simulink model "PB"  (R2025b)
settings: Solver=FixedStepAuto  StartTime=0.0  StopTime=inf  FixedStep=1E-2  RelTol=1e-3
libraries: aerolibanimutils x1
settings Model: Creator=abstract  LastModifiedBy=abstract

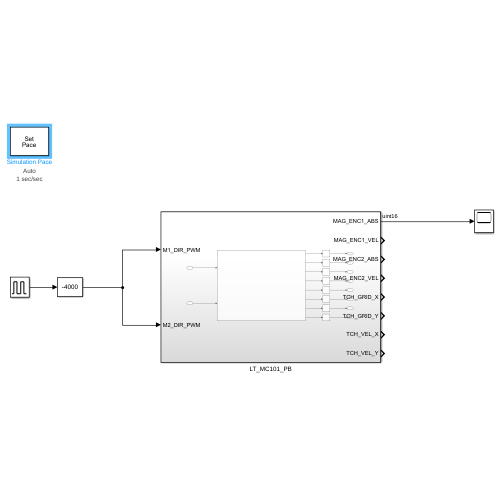
[thumbnail: Simulink's stored preview of the top-level diagram]
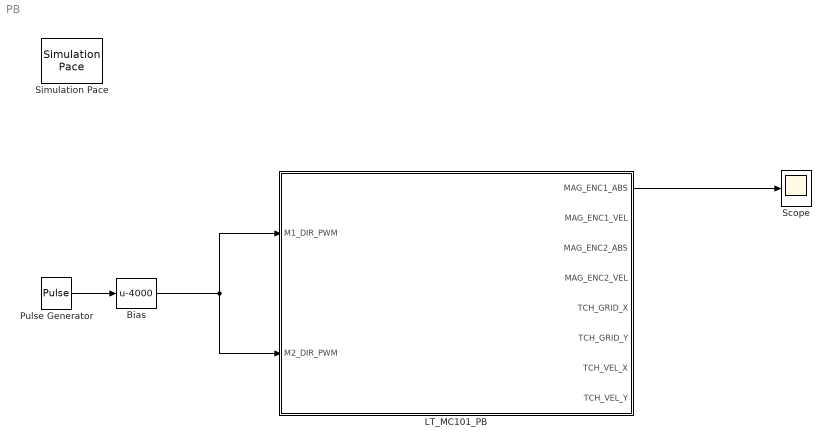
== system PB ==
  Bias : Bias  Bias=-4000  SaturateOnIntegerOverflow=off
  LT_MC101_PB : Subsystem
  Pulse Generator : DiscretePulseGenerator  PulseType=Time based  Amplitude=8000  Period=1  PulseWidth=50
  Scope : Scope
      settings: ActiveDisplayYMinimum=-62.499999999999986  ActiveDisplayYMaximum=562.5
  Simulation Pace : aerolibanimutils/Simulation Pace  SimulationPace=1  SleepMode=Auto  OutputPaceError=off  SampleTime=-1
  wires:
  Pulse Generator/1 -> Bias/1
  LT_MC101_PB/1(MAG_ENC1_ABS) -> Scope/1
  Bias/1 -> LT_MC101_PB/2(M2_DIR_PWM), LT_MC101_PB/1(M1_DIR_PWM)

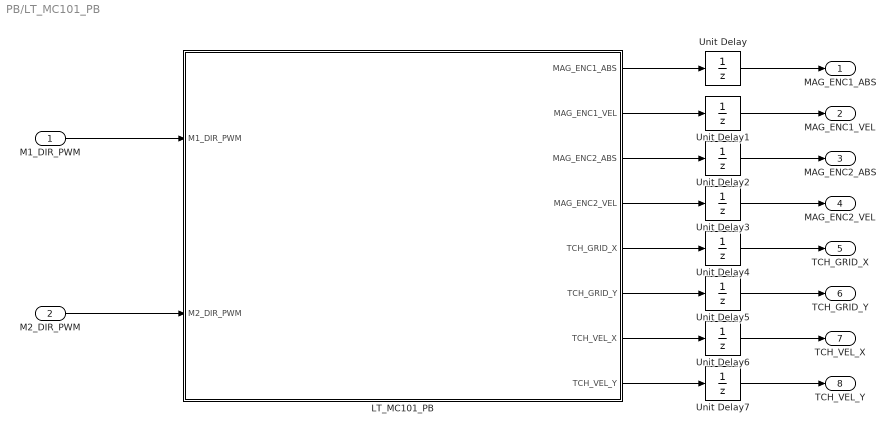
== system PB/LT_MC101_PB ==
  M1_DIR_PWM : Inport
  M2_DIR_PWM : Inport  Port=2
  LT_MC101_PB : MATLAB Function  TreatAsAtomicUnit=on
  Unit Delay{,1..7} (8 alike) : UnitDelay  SampleTime=-1  HasFrameUpgradeWarning=on
  MAG_ENC1_ABS : Outport  OutDataTypeStr=uint16
  MAG_ENC1_VEL : Outport  Port=2  OutDataTypeStr=single
  MAG_ENC2_ABS : Outport  Port=3  OutDataTypeStr=uint16
  MAG_ENC2_VEL : Outport  Port=4  OutDataTypeStr=single
  TCH_GRID_X : Outport  Port=5  OutDataTypeStr=single
  TCH_GRID_Y : Outport  Port=6  OutDataTypeStr=single
  TCH_VEL_X : Outport  Port=7  OutDataTypeStr=single
  TCH_VEL_Y : Outport  Port=8  OutDataTypeStr=single
  wires:
  LT_MC101_PB/3(MAG_ENC2_ABS) -> Unit Delay2/1
  M2_DIR_PWM/1 -> LT_MC101_PB/2(M2_DIR_PWM)
  LT_MC101_PB/7(TCH_VEL_X) -> Unit Delay6/1
  LT_MC101_PB/4(MAG_ENC2_VEL) -> Unit Delay3/1
  LT_MC101_PB/8(TCH_VEL_Y) -> Unit Delay7/1
  M1_DIR_PWM/1 -> LT_MC101_PB/1(M1_DIR_PWM)
  LT_MC101_PB/6(TCH_GRID_Y) -> Unit Delay5/1
  LT_MC101_PB/5(TCH_GRID_X) -> Unit Delay4/1
  LT_MC101_PB/1(MAG_ENC1_ABS) -> Unit Delay/1
  LT_MC101_PB/2(MAG_ENC1_VEL) -> Unit Delay1/1
  Unit Delay/1 -> MAG_ENC1_ABS/1
  Unit Delay1/1 -> MAG_ENC1_VEL/1
  Unit Delay2/1 -> MAG_ENC2_ABS/1
  Unit Delay3/1 -> MAG_ENC2_VEL/1
  Unit Delay6/1 -> TCH_VEL_X/1
  Unit Delay4/1 -> TCH_GRID_X/1
  Unit Delay5/1 -> TCH_GRID_Y/1
  Unit Delay7/1 -> TCH_VEL_Y/1

== matlab function PB/LT_MC101_PB/LT_MC101_PB ==
  data: MAG_ENC1_ABS output; MAG_ENC1_VEL output; M1_DIR_PWM input; MAG_ENC2_ABS output; MAG_ENC2_VEL output; M2_DIR_PWM input; TCH_GRID_X output; TCH_GRID_Y output; TCH_VEL_X output; TCH_VEL_Y output
function [MAG_ENC1_ABS, MAG_ENC1_VEL, MAG_ENC2_ABS, MAG_ENC2_VEL, TCH_GRID_X, TCH_GRID_Y, TCH_VEL_X, TCH_VEL_Y] = LT_MC101_PB(M1_DIR_PWM, M2_DIR_PWM)

Set_PB_Mx(int16(M1_DIR_PWM), int16(M2_DIR_PWM));

[MAG_ENC1_ABS, MAG_ENC1_VEL, MAG_ENC2_ABS, MAG_ENC2_VEL, TCH_GRID_X, TCH_GRID_Y, TCH_VEL_X, TCH_VEL_Y] = Get_PB_State();
